simulink model "observador_project_21_a"  (R2021a)
settings: Solver=ode4  StartTime=0.0  StopTime=10  FixedStep=0.01  RelTol=1e-3
values from neighbouring files (symbols this model uses):
  A = [-Ra/La -Kg/(Kt*La) ... (first row only)    [observador.m]    (also in observador_arduino.m)
  b = [1/La ; 0]    [observador.m]
  c = [0 1]    [observador.m]
  ki_1 = valid_ki(1)    [observador.m]
  l = double([sol.l_1;sol.l_2])    [observador.m]
settings Model: Creator=Guilherme  LastModifiedBy=Guilherme
settings DebuggingCC: UnconnectedInputMsg=none  UnconnectedOutputMsg=none  UnconnectedLineMsg=none
settings ModelReferenceCC: EnableRefExpFcnMdlSchedulingChecks=off
settings RTWCC: Description=Generic Real-Time Target  GPUComputeCapability=5.0  DLArmComputeVersion=20.02.1

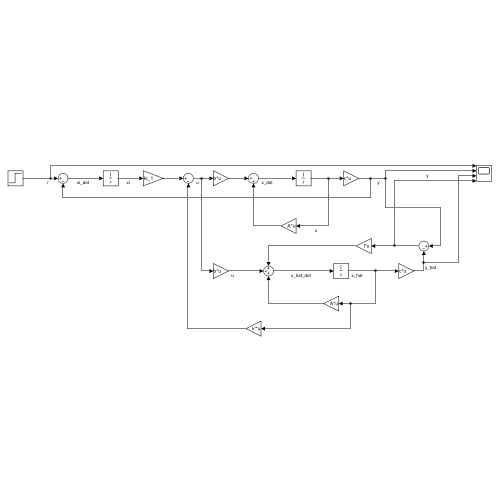
[thumbnail: Simulink's stored preview of the top-level diagram]
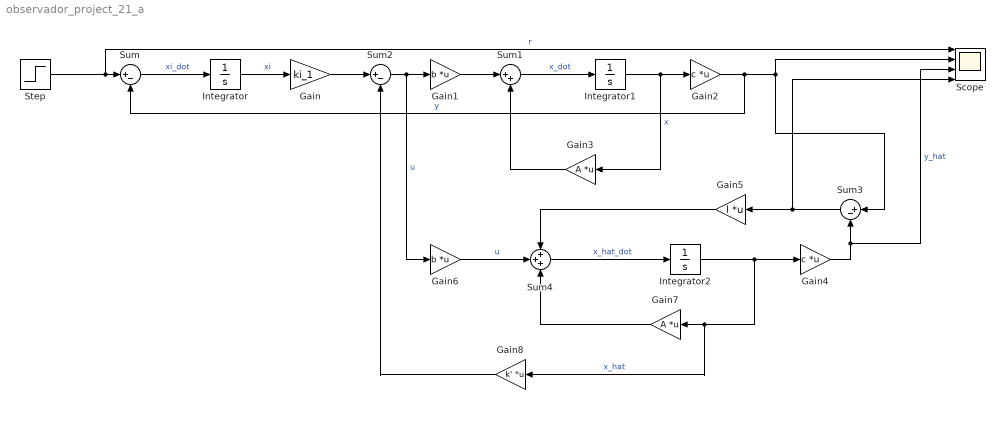
== system observador_project_21_a ==
  Gain : Gain  Gain=ki_1
  Gain1 : Gain  Gain=b  Multiplication=Matrix(K*u)
  Gain2 : Gain  Gain=c  Multiplication=Matrix(K*u)
  Gain3 : Gain  Gain=A  Multiplication=Matrix(K*u)
  Gain4 : Gain  Gain=c  Multiplication=Matrix(K*u)
  Gain5 : Gain  Gain=l  Multiplication=Matrix(K*u)
  Gain6 : Gain  Gain=b  Multiplication=Matrix(K*u)
  Gain7 : Gain  Gain=A  Multiplication=Matrix(K*u)
  Gain8 : Gain  Gain=k'  Multiplication=Matrix(K*u)
  Integrator : Integrator
  Integrator1 : Integrator
  Integrator2 : Integrator  InitialCondition=2
  Scope : Scope  NumInputPorts=4
  Step : Step  Time=0.1  Before=5  After=13  SampleTime=0
  Sum : Sum  Inputs=|+-
  Sum1 : Sum  Inputs=|++
  Sum2 : Sum  Inputs=|+-
  Sum3 : Sum  Inputs=|+-
  Sum4 : Sum  Inputs=+++
  wires:
  Step/1 -> Scope/1, Sum/1  "r"
  Sum/1 -> Integrator/1  "xi_dot"
  Integrator/1 -> Gain/1  "xi"
  Gain/1 -> Sum2/1
  Sum2/1 -> Gain6/1, Gain1/1  "u"
  Gain1/1 -> Sum1/1
  Sum1/1 -> Integrator1/1  "x_dot"
  Integrator1/1 -> Gain3/1, Gain2/1  "x"
  Gain2/1 -> Sum3/1, Scope/2, Sum/2  "y"
  Gain3/1 -> Sum1/2
  Gain4/1 -> Scope/3, Sum3/2  "y_hat"
  Sum3/1 -> Scope/4, Gain5/1
  Gain6/1 -> Sum4/2  "u"
  Gain5/1 -> Sum4/1
  Integrator2/1 -> Gain8/1, Gain7/1, Gain4/1  "x_hat"
  Sum4/1 -> Integrator2/1  "x_hat_dot"
  Gain7/1 -> Sum4/3
  Gain8/1 -> Sum2/2
